simulink library "gravityGrad_Lib"  (R2018b)
settings: Solver=VariableStepAuto  StartTime=0.0  StopTime=10.0  RelTol=1e-3
libraries: aerolibutil x1
settings Model: Creator=im11  LastModifiedBy=IvanMachuca

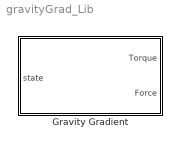
== system gravityGrad_Lib ==
  Gravity Gradient : Subsystem

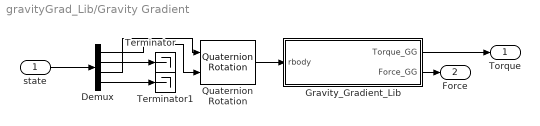
== system gravityGrad_Lib/Gravity Gradient ==
  state : Inport
  Demux : Demux  Outputs=[3 3 4 3]
  "Gravity_Gradient_Lib " : MATLAB Function  TreatAsAtomicUnit=on
  Quaternion Rotation : aerolibutil/Quaternion Rotation
  Terminator : Terminator
  Terminator1 : Terminator
  Torque : Outport
  Force : Outport  Port=2
  wires:
  "Gravity_Gradient_Lib "/1(Torque_GG) -> Torque/1
  "Gravity_Gradient_Lib "/2(Force_GG) -> Force/1
  state/1 -> Demux/1
  Demux/4 -> Terminator1/1
  Demux/2 -> Terminator/1
  Quaternion Rotation/1 -> "Gravity_Gradient_Lib "/1(rbody)
  Demux/1 -> Quaternion Rotation/2
  Demux/3 -> Quaternion Rotation/1

== matlab function gravityGrad_Lib/Gravity Gradient/Gravity_Gradient_Lib  ==
  data: rbody input; Torque_GG output; Force_GG output; simParams parameter
function [Torque_GG,Force_GG]  = GravityG(rbody,simParams)
%r_eci is the position vector in the reci coord frame in meters
%J is the moment of inertia
%q is the unit quaternion 
%This will output the gravity gradient torques from the initial position
%and torques

J = simParams.scParams.J;

rbody = rbody*1000; %converting to meters
%Eul = quatern2euler(q);
%Eul = quat2angle(q);
%Eul(1) = theta,Eul(2) = phi, Eul(3) = psi
%[DCM] = my_quat2dcm_last(q);

mu = 3.986004418e14; % in m^3/s^2
Ro = sqrt(rbody(1)^2+rbody(2)^2+rbody(3)^2);%in meters
L = 30e-2;%Longest length of CubeSat in m

a   = rbody;
b   = J*rbody;
axb = skew(a)*b;

%Torque will be in units of N-m This if we wanted to do it with euler
%angles
%Tx = 3*mu/(2*Ro^3)*(J(3,3)-J(2,2))*sin(2*Eul(2))*cos(Eul(1))^2;
%Ty = 3*mu/(2*Ro^3)*(J(3,3)-J(1,1))*sin(2*Eul(1))*cos(Eul(2))^2;
%Tz = 3*mu/(2*Ro^3)*(J(1,1)-J(2,2))*sin(2*Eul(1))*cos(Eul(2))^2;

%This equation (4.8.8) is from Spacecraft Dynamics and Control using DCM
% Tx = 3*mu/(2*Ro^3)*(J(3,3)-J(2,2))*DCM(2,3)*DCM(3,3);
% Ty = -3*mu/(2*Ro^3)*(J(3,3)-J(1,1))*DCM(1,3)*DCM(3,3);
% Tz = -3*mu/(2*Ro^3)*(J(1,1)-J(2,2))*DCM(1,3)*DCM(2,3);

Torque_GG = 3*mu/(norm(a)^5)*axb;%N-m
Force_GG = Torque_GG/L; %N


end
